simulink model "System"  (R2024a)
settings: Solver=VariableStepAuto  StartTime=0.0  StopTime=100  RelTol=1e-3
settings Model: Creator=Ashley  LastModifiedBy=Ashley

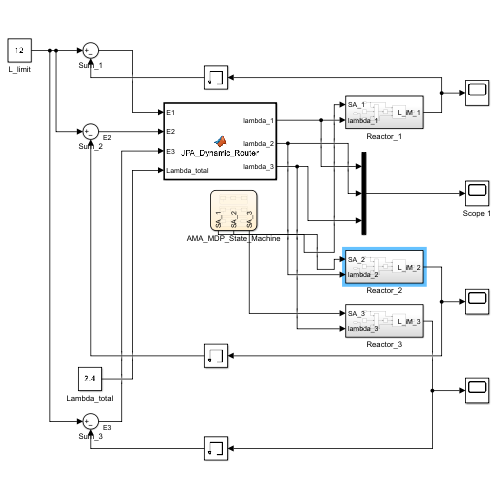
[thumbnail: Simulink's stored preview of the top-level diagram]
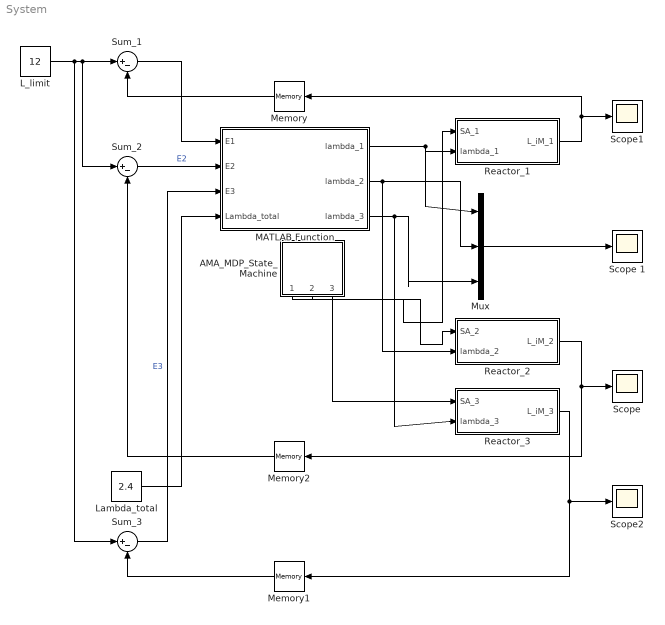
== system System ==
  AMA_MDP_State_Machine : Stateflow chart  TreatAsAtomicUnit=on
      settings: PortSchema="{\"entries\":[{\"content\":{\"sides\":[{\"content\":{},\"type\":\"ConnectorPlacement.EquallySpacedRectSide\",\"uuid\":\"7d3b9e99-ba35-4892-834a-debb18a64ce4\"},{\"content\":{\"side\":\"RIGHT\"},\"type\":\"ConnectorPlacement.EquallySpacedRectSide\",\"uuid\":\"bc62a211-1319-430c-90ce-06923850d148\"},{\"content\":{\"side\":\"TOP\"},\"type\":\"ConnectorPlacement.EquallySpacedRectSide\",\"uuid\":\"45f80e8b-ba38-4084-bd89-f1d64e97c6dd\"},{\"content\":{\"connectorIds\":[\"Out1\",\"Out2\",\"Out3\"],\"side\":\"BOTTOM\"},\"type\":\"ConnectorPlacement.EquallySpacedRectSide\",\"uuid\":\"96dac4f4-2c83-4a2d-a846-9b1ce2faefc2\"}]},\"type\":\"ConnectorPlacement.EquallySpacedConnector\",\"uuid\":\"ded2ea34-cce7-4828-a32f-28bcd15fcca8\"}],\"packageUris\":[\"http://schema.mathworks.com/mf0/Connector/R2020b\"],\"version\":\"1.0\"}"
  L_limit : Constant  Value=12
  Lambda_total : Constant  Value=2.4
  MATLAB Function : MATLAB Function  TreatAsAtomicUnit=on
  Memory : Memory
  Memory1 : Memory
  Memory2 : Memory
  Mux : Mux  Inputs=3
  Reactor_1 : Subsystem
  Reactor_2 : Subsystem
  Reactor_3 : Subsystem
  Scope : Scope
  Scope 1 : Scope
  Scope1 : Scope
  Scope2 : Scope
  Sum_1 : Sum  Inputs=|+-
  Sum_2 : Sum  Inputs=|+-
  Sum_3 : Sum  Inputs=|+-
  wires:
  AMA_MDP_State_Machine/3(SA_3) -> Reactor_3/1(SA_3)
  L_limit/1 -> Sum_1/1, Sum_2/1, Sum_3/1
  Sum_1/1 -> MATLAB Function/1(E1)
  Sum_2/1 -> MATLAB Function/2(E2)  "E2"
  Lambda_total/1 -> MATLAB Function/4(Lambda_total)
  AMA_MDP_State_Machine/2(SA_2) -> Reactor_2/1(SA_2)
  Sum_3/1 -> MATLAB Function/3(E3)  "E3"
  Memory/1 -> Sum_1/2
  MATLAB Function/2(lambda_2) -> Mux/2, Reactor_2/2(lambda_2)
  AMA_MDP_State_Machine/1(SA_1) -> Reactor_1/1(SA_1)
  Reactor_2/1(L_iM_2) -> Scope/1, Memory2/1
  Mux/1 -> Scope 1/1
  Memory2/1 -> Sum_2/2
  Memory1/1 -> Sum_3/2
  MATLAB Function/1(lambda_1) -> Mux/1, Reactor_1/2(lambda_1)
  Reactor_1/1(L_iM_1) -> Memory/1, Scope1/1
  MATLAB Function/3(lambda_3) -> Mux/3, Reactor_3/2(lambda_3)
  Reactor_3/1(L_iM_3) -> Scope2/1, Memory1/1

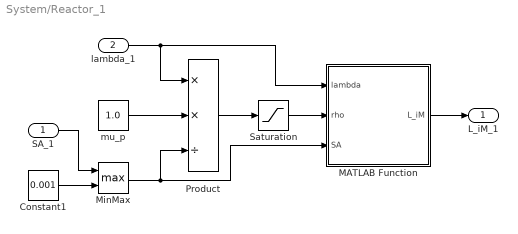
== system System/Reactor_1 ==
  SA_1 : Inport
  lambda_1 : Inport  Port=2
  Constant1 : Constant  Value=0.001
  MATLAB Function : MATLAB Function  TreatAsAtomicUnit=on
  MinMax : MinMax  Function=max  Inputs=2
  Product : Product  Inputs=**/
  Saturation : Saturate  UpperLimit=0.99  LowerLimit=0
  mu_p : Constant  Value=1.0
  L_iM_1 : Outport
  wires:
  SA_1/1 -> MinMax/1
  mu_p/1 -> Product/2
  Constant1/1 -> MinMax/2
  lambda_1/1 -> Product/1, MATLAB Function/1(lambda)
  MinMax/1 -> MATLAB Function/3(SA), Product/3
  MATLAB Function/1(L_iM) -> L_iM_1/1
  Saturation/1 -> MATLAB Function/2(rho)
  Product/1 -> Saturation/1

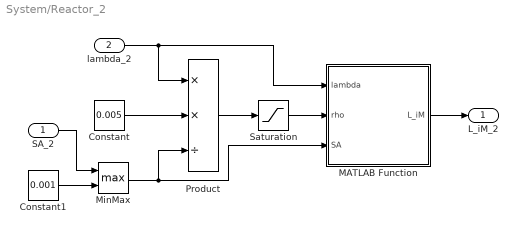
== system System/Reactor_2 ==
  SA_2 : Inport
  lambda_2 : Inport  Port=2
  Constant : Constant  Value=0.005
  Constant1 : Constant  Value=0.001
  MATLAB Function : MATLAB Function  TreatAsAtomicUnit=on
  MinMax : MinMax  Function=max  Inputs=2
  Product : Product  Inputs=**/
  Saturation : Saturate  UpperLimit=0.99  LowerLimit=0
  L_iM_2 : Outport
  wires:
  SA_2/1 -> MinMax/1
  Constant/1 -> Product/2
  Constant1/1 -> MinMax/2
  lambda_2/1 -> Product/1, MATLAB Function/1(lambda)
  MinMax/1 -> MATLAB Function/3(SA), Product/3
  MATLAB Function/1(L_iM) -> L_iM_2/1
  Saturation/1 -> MATLAB Function/2(rho)
  Product/1 -> Saturation/1

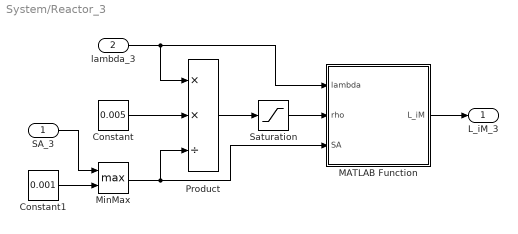
== system System/Reactor_3 ==
  SA_3 : Inport
  lambda_3 : Inport  Port=2
  Constant : Constant  Value=0.005
  Constant1 : Constant  Value=0.001
  MATLAB Function : MATLAB Function  TreatAsAtomicUnit=on
  MinMax : MinMax  Function=max  Inputs=2
  Product : Product  Inputs=**/
  Saturation : Saturate  UpperLimit=0.99  LowerLimit=0
  L_iM_3 : Outport
  wires:
  SA_3/1 -> MinMax/1
  Constant/1 -> Product/2
  Constant1/1 -> MinMax/2
  lambda_3/1 -> Product/1, MATLAB Function/1(lambda)
  MinMax/1 -> MATLAB Function/3(SA), Product/3
  MATLAB Function/1(L_iM) -> L_iM_3/1
  Saturation/1 -> MATLAB Function/2(rho)
  Product/1 -> Saturation/1

== matlab function System/Reactor_3/MATLAB Function ==
  data: lambda input; L_iM output; rho input; SA input
function L_iM = calculate_LeadTime(lambda, rho, SA)
    % 工艺常量设定
    mu_p = 1.0;   
    mu_q = 5.0;    
    r_i = 1.0;   
    z_d = 1.96;  

    % 物理防错机制：如果设备严重故障（SA极低），物理上等同于停工
    if SA < 0.1
        L_iM = 9999; % 强制赋予一个极大的提前期，瞬间引爆报警机制！
    else
        % 正常/退化时的公式计算
        linear_term = r_i * (mu_q + mu_p);
        queue_term = (lambda * rho * SA) / (2 * (1 - rho));
        L_iM = linear_term + z_d * sqrt(SA + queue_term);
    end
end

== matlab function System/Reactor_2/MATLAB Function ==
  data: lambda input; L_iM output; rho input; SA input
function L_iM = calculate_LeadTime(lambda, rho, SA)
    % 工艺常量设定
    mu_p = 1.0;   
    mu_q = 5.0;    
    r_i = 1.0;   
    z_d = 1.96;  

    % 物理防错机制：如果设备严重故障（SA极低），物理上等同于停工
    if SA < 0.1
        L_iM = 9999; % 强制赋予一个极大的提前期，瞬间引爆报警机制！
    else
        % 正常/退化时的公式计算
        linear_term = r_i * (mu_q + mu_p);
        queue_term = (lambda * rho * SA) / (2 * (1 - rho));
        L_iM = linear_term + z_d * sqrt(SA + queue_term);
    end
end

== matlab function System/MATLAB Function ==
  data: E1 input; lambda_1 output; E2 input; E3 input; Lambda_total input; lambda_2 output; lambda_3 output
function [lambda_1, lambda_2, lambda_3] = JPA_Dynamic_Router(E1, E2, E3, Lambda_total)
    % 默认状态：如果所有反应釜提前期都健康（E >= 0），则将总流率平均分配
    lambda_1 = Lambda_total / 3;
    lambda_2 = Lambda_total / 3;
    lambda_3 = Lambda_total / 3;

    % 动态路由逻辑：检测是否有反应釜提前期超标 (E < 0 表示当前提前期超出了容差)
    % 优先级可以根据实际业务调整，这里采用互斥的 elseif 结构
    
    if E2 < 0
        % 反应釜 2 告急：切断分配，由 1 和 3 平摊
        lambda_2 = 0;
        lambda_1 = Lambda_total / 2;
        lambda_3 = Lambda_total / 2;
        
    elseif E1 < 0
        % 反应釜 1 告急：切断分配，由 2 和 3 平摊
        lambda_1 = 0;
        lambda_2 = Lambda_total / 2;
        lambda_3 = Lambda_total / 2;
        
    elseif E3 < 0
        % 反应釜 3 告急：切断分配，由 1 和 2 平摊
        lambda_3 = 0;
        lambda_1 = Lambda_total / 2;
        lambda_2 = Lambda_total / 2;
    end
    
    % 注意：如果真实车间有两个同时告急，代码可以进一步扩展（比如全部分给剩下的1个），
    % 本代码满足您当前单点故障注入的仿真验证需求。
end

== stateflow chart System/AMA_MDP_State_Machine ==
  state Reactor3_State [parallel]
    settings: executionOrder=3
    state Normal_3
      en: SA_3 = 1.0;
    state Degraded_3
      en: SA_3 = 0.7;
    state Maint_3
      en: SA_3 = 0.001;
    Normal_3 -> Degraded_3 : after(30, sec)
    Degraded_3 -> Maint_3 : after(20, sec)
    (default) -> Normal_3
  state Reactor2_State [parallel]
    settings: executionOrder=2
    state Normal_2
      en: SA_2 = 1.0;
    state Degraded_2
      en: SA_2 = 0.7;
    state Maint_2
      en: SA_2 = 0.001;
    Normal_2 -> Degraded_2 : after(30, sec)
    Degraded_2 -> Maint_2 : after(20, sec)
    (default) -> Normal_2
  state Reactor1_State [parallel]
    settings: executionOrder=1
    state Normal_1
      en: SA_1 = 1.0;
    state Degraded_1
      en: SA_1 = 0.7;
    state Maint_1
      en: SA_1 = 0.001;
    Normal_1 -> Degraded_1 : after(30, sec)
    Degraded_1 -> Maint_1 : after(20, sec)
    (default) -> Normal_1
  data: SA_1 output; SA_2 output; SA_3 output

== matlab function System/Reactor_1/MATLAB Function ==
  data: lambda input; L_iM output; rho input; SA input
function L_iM = calculate_LeadTime(lambda, rho, SA)
    % 工艺常量设定
    mu_p = 1.0;   
    mu_q = 5.0;    
    r_i = 1.0;   
    z_d = 1.96;  

    % 物理防错机制：如果设备严重故障（SA极低），物理上等同于停工
    if SA < 0.1
        L_iM = 9999; % 强制赋予一个极大的提前期，瞬间引爆报警机制！
    else
        % 正常/退化时的公式计算
        linear_term = r_i * (mu_q + mu_p);
        queue_term = (lambda * rho * SA) / (2 * (1 - rho));
        L_iM = linear_term + z_d * sqrt(SA + queue_term);
    end
end
